simulink model "AAI_prev"  (R2022a)
settings: Solver=FixedStepAuto  StartTime=0.0  StopTime=10.0  FixedStep=1e-3  RelTol=1e-3  EnableMultiTasking=on
undefined symbols (not defined in the file): D0, D10, D11, D12, D13, D2, D4, D5, D6, D7, D8, D9, PTA0, PTA2, PTB23, PTB9, PTC16, PTC2, PTC3, PTC4, PTD0, PTD1, PTD2, PTD3
libraries: frdmk64flib x14
settings Model: ExtModeTrigDuration=5  Creator=jacqu  LastModifiedBy=asus
settings OptimizationCC: EnhancedBackFolding=on  PassReuseOutputArgsAs=Individual arguments  ZeroExternalMemoryAtStartup=off  ZeroInternalMemoryAtStartup=off  MaxStackSize=64  OptimizeBlockOrder=speed  DifferentSizesBufferReuse=on  OptimizationCustomize=off  EfficientTunableParamExpr=on
settings DebuggingCC: ParameterTunabilityLossMsg=error
settings HardwareCC: ProdBitPerPointer=32  ProdBitPerSizeT=32  ProdBitPerPtrDiffT=32  ProdLargestAtomicInteger=Long  ProdLargestAtomicFloat=Double  ProdWordSize=32  ProdHWDeviceType=ARM Compatible->ARM Cortex
settings SFSimCC: MATLABDynamicMemAlloc=off
settings RTWCC: SystemTargetFile=ert.tlc  HardwareBoard=NXP FRDM-K64F  TLCOptions="-aInlineSetEventsForThisBaseRateFcn=TLC_FALSE -aSuppressMultiTaskScheduler=TLC_FALSE  -aRateBasedStepFcn=0"  TemplateMakefile=ert_default_tmf  Toolchain=GNU Tools for ARM Embedded Processors
settings CodeAppCC: ForceParamTrailComments=on  IgnoreCustomStorageClasses=off  OperatorAnnotations=on  SimulinkDataObjDesc=on  SFDataObjDesc=on  InsertBlockDesc=on
settings ERTTargetCC: ExtModeTransport=4  ExtModeMexFile=sendToCommService

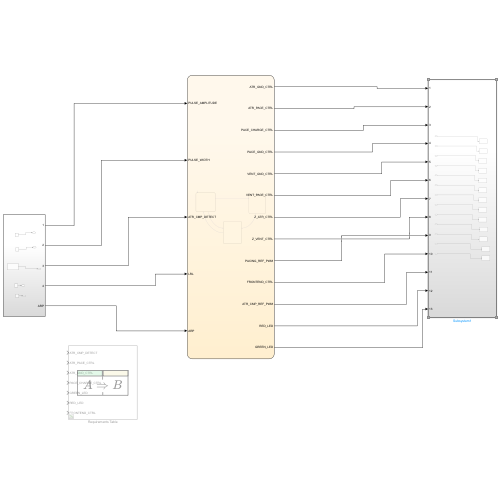
[thumbnail: Simulink's stored preview of the top-level diagram]
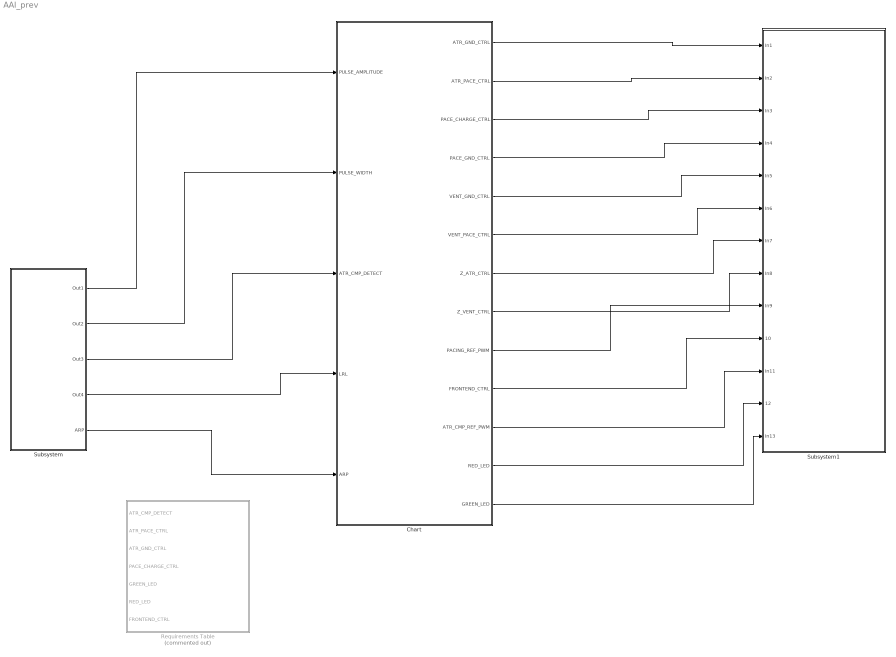
== system AAI_prev ==
  Chart : Stateflow chart  TreatAsAtomicUnit=on
  Requirements Table : Requirements Table  Commented=on  TreatAsAtomicUnit=on
  Subsystem : Subsystem
  Subsystem1 : Subsystem
  wires:
  Subsystem/4(Out4) -> Chart/4(LRL)
  Subsystem/1(Out1) -> Chart/1(PULSE_AMPLITUDE)
  Subsystem/2(Out2) -> Chart/2(PULSE_WIDTH)
  Subsystem/3(Out3) -> Chart/3(ATR_CMP_DETECT)
  Chart/1(ATR_GND_CTRL) -> Subsystem1/1(In1)
  Chart/2(ATR_PACE_CTRL) -> Subsystem1/2(In2)
  Chart/3(PACE_CHARGE_CTRL) -> Subsystem1/3(In3)
  Chart/4(PACE_GND_CTRL) -> Subsystem1/4(In4)
  Chart/5(VENT_GND_CTRL) -> Subsystem1/5(In5)
  Chart/6(VENT_PACE_CTRL) -> Subsystem1/6(In6)
  Chart/7(Z_ATR_CTRL) -> Subsystem1/7(In7)
  Chart/8(Z_VENT_CTRL) -> Subsystem1/8(In8)
  Chart/9(PACING_REF_PWM) -> Subsystem1/9(In9)
  Chart/10(FRONTEND_CTRL) -> Subsystem1/10(10)
  Chart/11(ATR_CMP_REF_PWM) -> Subsystem1/11(In11)
  Chart/12(RED_LED) -> Subsystem1/12(12)
  Chart/13(GREEN_LED) -> Subsystem1/13(In13)
  Subsystem/5(ARP) -> Chart/5(ARP)

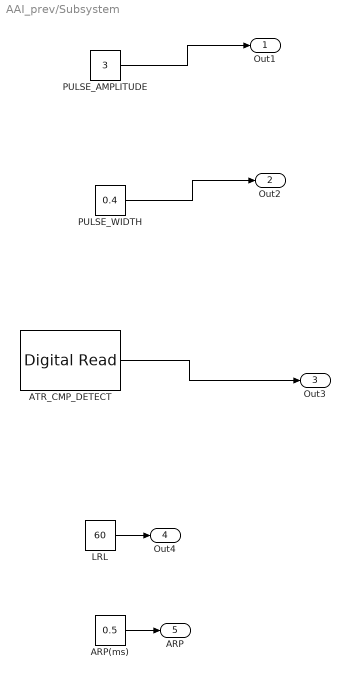
== system AAI_prev/Subsystem ==
  ARP(ms) : Constant  Value=0.5
  ATR_CMP_DETECT : frdmk64flib/Digital Read  Whichpin=PTC16 (D0)  SampleTime=-1
  LRL : Constant  Value=60
  PULSE_AMPLITUDE : Constant  Value=3
  PULSE_WIDTH : Constant  Value=0.4
  Out1 : Outport
  Out2 : Outport  Port=2
  Out3 : Outport  Port=3
  Out4 : Outport  Port=4
  ARP : Outport  Port=5
  wires:
  PULSE_AMPLITUDE/1 -> Out1/1
  PULSE_WIDTH/1 -> Out2/1
  ATR_CMP_DETECT/1 -> Out3/1
  LRL/1 -> Out4/1
  ARP(ms)/1 -> ARP/1

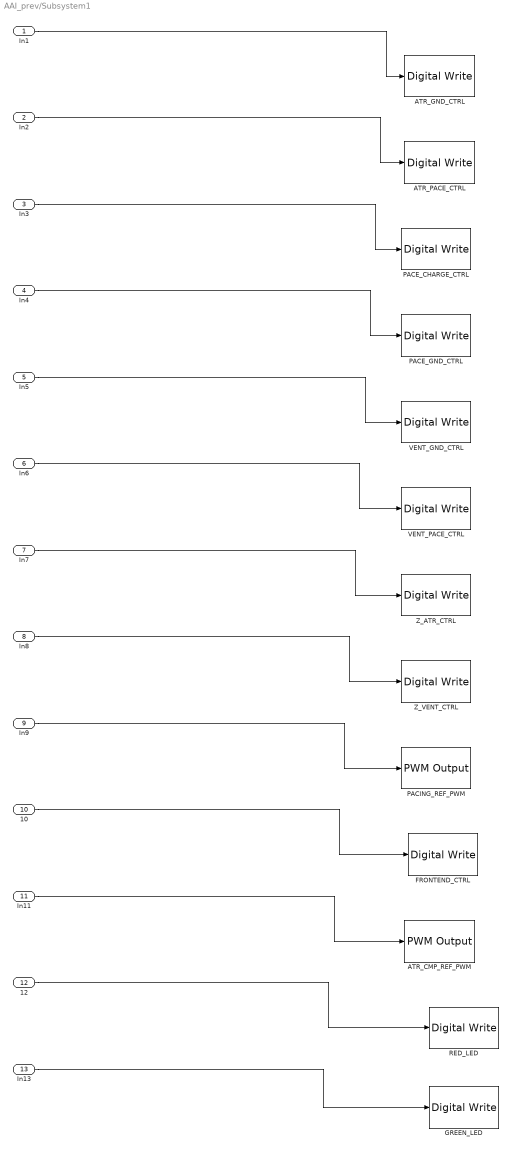
== system AAI_prev/Subsystem1 ==
  In1 : Inport
  In2 : Inport  Port=2
  In3 : Inport  Port=3
  In4 : Inport  Port=4
  In5 : Inport  Port=5
  In6 : Inport  Port=6
  In7 : Inport  Port=7
  In8 : Inport  Port=8
  In9 : Inport  Port=9
  10 : Inport  Port=10
  In11 : Inport  Port=11
  12 : Inport  Port=12
  In13 : Inport  Port=13
  " ATR_CMP_REF_PWM" : frdmk64flib/PWM Output  Whichpin=PTC2 (D6)  InitialFrequency=2000  InitialDutyCycle=0
  " PACING_REF_PWM" : frdmk64flib/PWM Output  Whichpin=PTA2 (D5)  InitialFrequency=2000  InitialDutyCycle=0
  ATR_GND_CTRL : frdmk64flib/Digital Write  Whichpin=PTD2 (D11)
  ATR_PACE_CTRL : frdmk64flib/Digital Write  Whichpin=PTA0 (D8)
  FRONTEND_CTRL : frdmk64flib/Digital Write  Whichpin=PTD1 (D13)
  GREEN_LED : frdmk64flib/Digital Write  Whichpin=GREEN_LED
  PACE_CHARGE_CTRL : frdmk64flib/Digital Write  Whichpin=PTB9 (D2)
  PACE_GND_CTRL : frdmk64flib/Digital Write  Whichpin=PTD0 (D10)
  RED_LED : frdmk64flib/Digital Write  Whichpin=RED_LED
  VENT_GND_CTRL : frdmk64flib/Digital Write  Whichpin=PTD3 (D12)
  VENT_PACE_CTRL : frdmk64flib/Digital Write  Whichpin=PTC4 (D9)
  Z_ATR_CTRL : frdmk64flib/Digital Write  Whichpin=PTB23 (D4)
  Z_VENT_CTRL : frdmk64flib/Digital Write  Whichpin=PTC3 (D7)
  wires:
  In11/1 -> " ATR_CMP_REF_PWM"/1
  In2/1 -> ATR_PACE_CTRL/1
  In9/1 -> " PACING_REF_PWM"/1
  In3/1 -> PACE_CHARGE_CTRL/1
  In13/1 -> GREEN_LED/1
  In4/1 -> PACE_GND_CTRL/1
  In1/1 -> ATR_GND_CTRL/1
  10/1 -> FRONTEND_CTRL/1
  In7/1 -> Z_ATR_CTRL/1
  12/1 -> RED_LED/1
  In5/1 -> VENT_GND_CTRL/1
  In8/1 -> Z_VENT_CTRL/1
  In6/1 -> VENT_PACE_CTRL/1

== stateflow chart AAI_prev/Requirements Table ==
  (default) -> (junction 1073742813)
  (junction 1073742813) -> (junction 1073742814) : {
      | % SF_REQ_REV_07
      | }
  (junction 1073742814) -> (junction 1073742816) : {
      | % HEADER_ASSIGNMENTS
      |
      | }
  (junction 1073742816) -> (junction 1073742818) : {
      | % START_A_4
      | }
  (junction 1073742818) -> (junction 1073742820) : {
      | }
  (junction 1073742820) -> (junction 1073742822)
  (junction 1073742822) -> (junction 1073742824) : {
      | }
  (junction 1073742824) -> (junction 1073742826) : {
      | % END_A_4
      | }
  (junction 1073742826) -> (junction 1073742828) : {
      | % START_R_1
      | }
  (junction 1073742828) -> (junction 1073742830) : {
      | }
  (junction 1073742830) -> (junction 1073742832) : {
      |
      |
      |
      |
      |
      |
      | }
  (junction 1073742832) -> (junction 1073742834) : {
      | }
  (junction 1073742834) -> (junction 1073742836) : {
      | % START_R_7
      | }
  (junction 1073742836) -> (junction 1073742838) : {
      | }
  (junction 1073742838) -> (junction 1073742840)
  (junction 1073742840) -> (junction 1073742842) [order 1] : [(prev(FRONTEND_CTRL)==true) && (prev(PACE_CHARGE_CTRL)==true) && (prev(ATR_PACE_CTRL)==false) && (prev(ATR_GND_CTRL)==true) && (prev(RED_LED)==false) && (prev(GREEN_LED)==false)]
  (junction 1073742840) -> (junction 1073742884) [order 2]
  (junction 1073742842) -> (junction 1073742844) : {
      |
      |
      |
      |
      |
      |
      | }
  (junction 1073742844) -> (junction 1073742846) : {
      | }
  (junction 1073742846) -> (junction 1073742848) : {
      | % START_R_10
      | }
  (junction 1073742848) -> (junction 1073742850) : {
      | }
  (junction 1073742850) -> (junction 1073742852)
  (junction 1073742852) -> (junction 1073742854) [order 1] : [(prev(ATR_CMP_DETECT)==true)]
  (junction 1073742852) -> (junction 1073742860) [order 2]
  (junction 1073742854) -> (junction 1073742856) : {
      | reqtable_postcondition((FRONTEND_CTRL==false) && (PACE_CHARGE_CTRL==false) && (ATR_PACE_CTRL==false) && (ATR_GND_CTRL == true) && (GREEN_LED==true), 'R:1.1.1');
      |
      |
      |
      |
      |
      |
      | }
  (junction 1073742856) -> (junction 1073742858) : {
      | }
  (junction 1073742858) -> (junction 1073742860)
  (junction 1073742860) -> (junction 1073742862)
  (junction 1073742862) -> (junction 1073742864) : {
      | % END_R_10
      | }
  (junction 1073742864) -> (junction 1073742866) : {
      | % START_R_13
      | }
  (junction 1073742866) -> (junction 1073742868) : {
      | }
  (junction 1073742868) -> (junction 1073742870)
  (junction 1073742870) -> (junction 1073742872) [order 1] : [duration((prev(ATR_CMP_DETECT)==false)) >= ((60000/LRL)-PULSE_WIDTH)/1000]
  (junction 1073742870) -> (junction 1073742878) [order 2]
  (junction 1073742872) -> (junction 1073742874) : {
      | reqtable_postcondition((FRONTEND_CTRL==true) && (PACE_CHARGE_CTRL==false) && (ATR_PACE_CTRL==true) && (ATR_GND_CTRL == false) && (RED_LED==true), 'R:1.1.2');
      |
      |
      |
      |
      |
      |
      | }
  (junction 1073742874) -> (junction 1073742876) : {
      | }
  (junction 1073742876) -> (junction 1073742878)
  (junction 1073742878) -> (junction 1073742880)
  (junction 1073742880) -> (junction 1073742882) : {
      | % END_R_13
      | }
  (junction 1073742882) -> (junction 1073742884)
  (junction 1073742884) -> (junction 1073742886)
  (junction 1073742886) -> (junction 1073742888) : {
      | % END_R_7
      | }
  (junction 1073742888) -> (junction 1073742890) : {
      | % START_R_16
      | }
  (junction 1073742890) -> (junction 1073742892) : {
      | }
  (junction 1073742892) -> (junction 1073742894)
  (junction 1073742894) -> (junction 1073742896) [order 1] : [(prev(FRONTEND_CTRL)==true) && (prev(PACE_CHARGE_CTRL)==false) && (prev(ATR_PACE_CTRL)==true) && (prev(ATR_GND_CTRL)==false) && (prev(RED_LED)==true) && (prev(GREEN_LED)==false)]
  (junction 1073742894) -> (junction 1073742938) [order 2]
  (junction 1073742896) -> (junction 1073742898) : {
      |
      |
      |
      |
      |
      |
      | }
  (junction 1073742898) -> (junction 1073742900) : {
      | }
  (junction 1073742900) -> (junction 1073742902) : {
      | % START_R_19
      | }
  (junction 1073742902) -> (junction 1073742904) : {
      | }
  (junction 1073742904) -> (junction 1073742906)
  (junction 1073742906) -> (junction 1073742908) [order 1] : [duration((prev(ATR_CMP_DETECT)==false)) >= (PULSE_WIDTH)/1000]
  (junction 1073742906) -> (junction 1073742914) [order 2]
  (junction 1073742908) -> (junction 1073742910) : {
      | reqtable_postcondition((FRONTEND_CTRL==true) && (PACE_CHARGE_CTRL==true) && (ATR_PACE_CTRL==false) && (ATR_GND_CTRL == true) && (RED_LED==false), 'R:1.2.1');
      |
      |
      |
      |
      |
      |
      | }
  (junction 1073742910) -> (junction 1073742912) : {
      | }
  (junction 1073742912) -> (junction 1073742914)
  (junction 1073742914) -> (junction 1073742916)
  (junction 1073742916) -> (junction 1073742918) : {
      | % END_R_19
      | }
  (junction 1073742918) -> (junction 1073742920) : {
      | % START_R_22
      | }
  (junction 1073742920) -> (junction 1073742922) : {
      | }
  (junction 1073742922) -> (junction 1073742924)
  (junction 1073742924) -> (junction 1073742926) [order 1] : [(prev(ATR_CMP_DETECT)==true)]
  (junction 1073742924) -> (junction 1073742932) [order 2]
  (junction 1073742926) -> (junction 1073742928) : {
      | reqtable_postcondition((FRONTEND_CTRL==false) && (PACE_CHARGE_CTRL==false) && (ATR_PACE_CTRL==false) && (ATR_GND_CTRL == true) && (GREEN_LED==true), 'R:1.2.2');
      |
      |
      |
      |
      |
      |
      | }
  (junction 1073742928) -> (junction 1073742930) : {
      | }
  (junction 1073742930) -> (junction 1073742932)
  (junction 1073742932) -> (junction 1073742934)
  (junction 1073742934) -> (junction 1073742936) : {
      | % END_R_22
      | }
  (junction 1073742936) -> (junction 1073742938)
  (junction 1073742938) -> (junction 1073742940)
  (junction 1073742940) -> (junction 1073742942) : {
      | % END_R_16
      | }
  (junction 1073742942) -> (junction 1073742944) : {
      | % START_R_25
      | }
  (junction 1073742944) -> (junction 1073742946) : {
      | }
  (junction 1073742946) -> (junction 1073742948)
  (junction 1073742948) -> (junction 1073742950) [order 1] : [(prev(FRONTEND_CTRL)==false) && (prev(PACE_CHARGE_CTRL)==false) && (prev(ATR_PACE_CTRL)==false) && (prev(ATR_GND_CTRL)==true) && (prev(GREEN_LED)==true)]
  (junction 1073742948) -> (junction 1073742956) [order 2]
  (junction 1073742950) -> (junction 1073742952) : {
      | reqtable_postcondition((FRONTEND_CTRL==true) && (PACE_CHARGE_CTRL==true) && (ATR_PACE_CTRL==false) && (ATR_GND_CTRL == true) && (GREEN_LED==false), 'R:1.3');
      |
      |
      |
      |
      |
      |
      | }
  (junction 1073742952) -> (junction 1073742954) : {
      | }
  (junction 1073742954) -> (junction 1073742956)
  (junction 1073742956) -> (junction 1073742958)
  (junction 1073742958) -> (junction 1073742960) : {
      | % END_R_25
      | }
  (junction 1073742960) -> (junction 1073742962) : {
      | % END_R_1
      | }
  data: ATR_CMP_DETECT input; PULSE_WIDTH constant double; LRL constant double; ATR_PACE_CTRL input; ATR_GND_CTRL input; PACE_CHARGE_CTRL input; GREEN_LED input; RED_LED input; FRONTEND_CTRL input

== stateflow chart AAI_prev/Chart ==
  state PACE_OFF
    entry:
    ATR_PACE_CTRL = 0
    VENT_PACE_CTRL = 0
    PACING_REF_PWM = 20*PULSE_AMPLITUDE
    PACE_CHARGE_CTRL = 1
    PACE_GND_CTRL = 1
    Z_ATR_CTRL = 0
    Z_VENT_CTRL = 0
    ATR_GND_CTRL = 1
    VENT_GND_CTRL = 0
    FRONTEND_CTRL = 1
    ATR_CMP_REF_PWM = 20*PULSE_AMPLITUDE
    % light indicators
    RED_LED = 0
    GREEN_LED = 0
  state PACE_ON
    entry:
    PACE_CHARGE_CTRL = 0
    PACE_GND_CTRL = 1
    ATR_PACE_CTRL = 1
    ATR_GND_CTRL = 0
    Z_ATR_CTRL = 0
    Z_VENT_CTRL = 0
    VENT_GND_CTRL = 0
    VENT_PACE_CTRL = 0
    % light indicator
    RED_LED = 1
  note: at paceon state, the system waits for the atr_cmp_detect signal to decide which
      | mode to go to . if atr_cmp_detect == 0, pace on. else, go refractory mode.
  note: when pacing, after the pulse width,
      | the mode would change to refractory mdoe
  state REFRACTORY
    entry:
    FRONTEND_CTRL = 0
    ATR_PACE_CTRL = 0
    ATR_GND_CTRL = 1
    PACING_REF_PWM = 20*PULSE_AMPLITUDE
    PACE_CHARGE_CTRL = 0
    PACE_GND_CTRL = 1
    % light indicator
    GREEN_LED = 1
  (default) -> PACE_OFF
  PACE_OFF -> PACE_ON [order 1] : [(ATR_CMP_DETECT == 0) && after((60000/LRL)-PULSE_WIDTH-ARP,msec)]
  PACE_ON -> REFRACTORY : [after(PULSE_WIDTH,msec)]
  REFRACTORY -> PACE_OFF : [after(ARP,msec)]
  PACE_OFF -> REFRACTORY [order 2] : [ATR_CMP_DETECT == 1]
  data: ATR_GND_CTRL output; ATR_PACE_CTRL output; PACE_CHARGE_CTRL output; PACE_GND_CTRL output; VENT_GND_CTRL output; VENT_PACE_CTRL output; Z_ATR_CTRL output; Z_VENT_CTRL output; PULSE_AMPLITUDE input; PACING_REF_PWM output; FRONTEND_CTRL output; ATR_CMP_REF_PWM output; RED_LED output; PULSE_WIDTH input; ATR_CMP_DETECT input; GREEN_LED output; LRL input; ARP input
